simulink model "Simulation"  (R2022b)
settings: Solver=ode1  StartTime=0.0  StopTime=Tf  FixedStep=t_step  RelTol=1e-3
undefined symbols (not defined in the file or in its folder): F, Im, Kd, Kp, kr, lx, ly, lz, mm, qt, rho, t_step
libraries: slpidlib x1
settings Model: Creator=vincenzo  LastModifiedBy=vincenzo

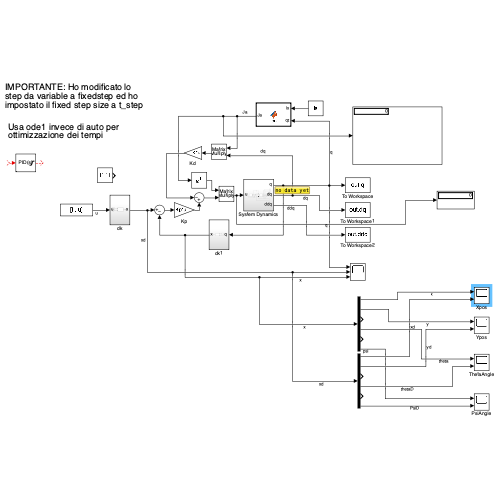
[thumbnail: Simulink's stored preview of the top-level diagram]
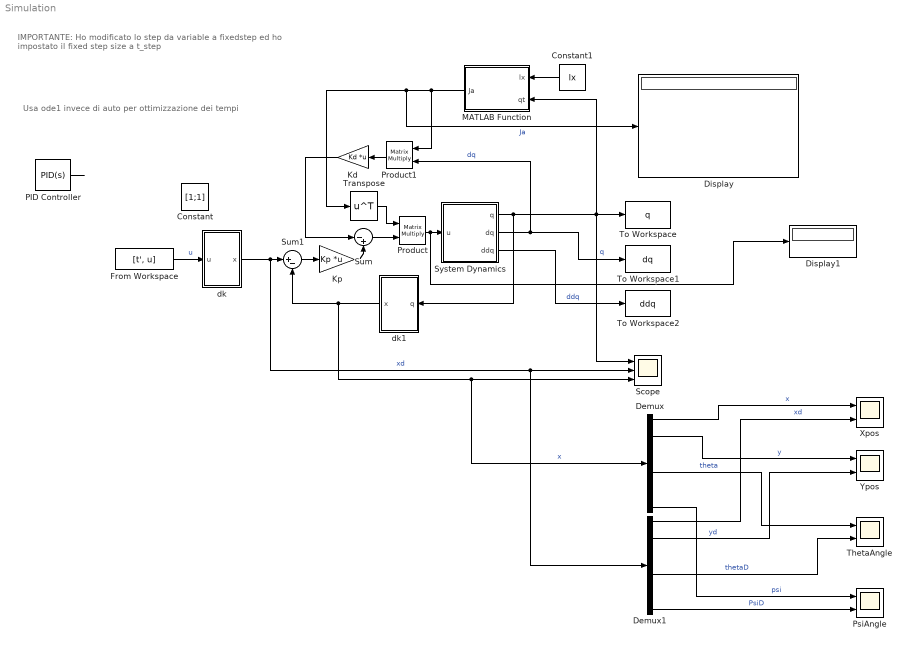
== system Simulation ==
  note: Usa ode1 invece di auto per ottimizzazione dei tempi
  note: IMPORTANTE: Ho modificato lo step da variable a fixedstep ed ho impostato il fixed step size a t_step
  Constant : Constant  Value=[1;1]
  Constant1 : Constant  Value=lx
  Demux : Demux  Outputs=6
  Demux1 : Demux  Outputs=6
  Display : Display
  Display1 : Display
  From Workspace : FromWorkspace  VariableName=[t', u]  OutDataTypeStr=double  SampleTime=t_step
  Kd : Gain  Gain=Kd  Multiplication=Matrix(K*u)
  Kp : Gain  Gain=Kp  Multiplication=Matrix(K*u)
  MATLAB Function : MATLAB Function  TreatAsAtomicUnit=on
  PID Controller : slpidlib/PID Controller  Controller=PID  Form=Parallel  TimeDomain=Continuous-time  UseExternalTs=off  SampleTime=-1  IntegratorMethod=Forward Euler  FilterMethod=Forward Euler  ControllerParametersSource=internal  P=1/100  I=0  UseKiTs=off  D=0  N=100  UseFilter=on  TunerSelectOption=Transfer Function Based (PID Tuner App)  InitialConditionSource=internal  InitialConditionForIntegrator=0  InitialConditionForFilter=0  DifferentiatorICPrevScaledInput=0  ExternalReset=none  TrackingMode=off  Kt=1  LimitOutput=on  SatLimitsSource=internal  UpperSaturationLimit=4.5  LowerSaturationLimit=-4.5  LinearizeAsGain=on  AntiWindupMode=clamping  Kb=1  LimitIntegrator=off  UpperIntegratorSaturationLimit=inf  LowerIntegratorSaturationLimit=-inf  POutMin=[]  POutMax=[]  IOutMin=[]  IOutMax=[]  DOutMin=[]  DOutMax=[]  NOutMin=[]  NOutMax=[]  SumOutMin=[]  SumOutMax=[]  SaturationOutMin=[]  SaturationOutMax=[]  PParamMin=[]  PParamMax=[]  IParamMin=[]  IParamMax=[]  DParamMin=[]  DParamMax=[]  NParamMin=[]  NParamMax=[]  KbParamMin=[]  KbParamMax=[]  KtParamMin=[]  KtParamMax=[]  KbOutMin=[]  KbOutMax=[]  KtOutMin=[]  KtOutMax=[]  IntegratorOutMin=[]  IntegratorOutMax=[]  FilterOutMin=[]  FilterOutMax=[]  SumI1OutMin=[]  SumI1OutMax=[]  SumI2OutMin=[]  SumI2OutMax=[]  SumI3OutMin=[]  SumI3OutMax=[]  SumI4OutMin=[]  SumI4OutMax=[]  SumDOutMin=[]  SumDOutMax=[]  DifferentiatorOutMin=[]  DifferentiatorOutMax=[]  FilterDiffOutCoefMin=[]  FilterDiffOutCoefMax=[]  ReciprocalOutMin=[]  ReciprocalOutMax=[]  SumDenOutMin=[]  SumDenOutMax=[]  SumNumOutMin=[]  SumNumOutMax=[]  DivideOutMin=[]  DivideOutMax=[]  UdiffTsProdOutMin=[]  UdiffTsProdOutMax=[]  NTsProdOutMin=[]  NTsProdOutMax=[]  UintegralTsProdOutMin=[]  UintegralTsProdOutMax=[]  UngainTsProdOutMin=[]  UngainTsProdOutMax=[]  ClampingZeroOutDataTypeStr=Inherit: Inherit via back propagation  ClampingZeroOutMin=[]  ClampingZeroOutMax=[]  FilterDenConstantOutDataTypeStr=Inherit: Inherit via back propagation  FilterDenConstantOutMin=[]  FilterDenConstantOutMax=[]  PCopyOutDataTypeStr=Inherit: Inherit via back propagation  PCopyOutMin=[]  PCopyOutMax=[]  NCopyOutDataTypeStr=Inherit: Inherit via back propagation  NCopyOutMin=[]  NCopyOutMax=[]  IntegratorContinuousStateAttributes=''  IntegratorStateMustResolveToSignalObject=off  IntegratorRTWStateStorageClass=Auto  FilterContinuousStateAttributes=''  FilterStateMustResolveToSignalObject=off  FilterRTWStateStorageClass=Auto  ParallelPVariant=InternalParameters  IdealPVariant=Disabled  IVariant=InternalParameters  DVariant=InternalParameters  IntegratorVariant=Continuous  SatVariant=Enabled  AWVariant=ContClampingParallel  PCopyVariant=Disabled  TRVariant=Disabled  FdbkBlocksVariant=Forward  IdealPFdbkVariant=Disabled  SatFdbkVariant=Disabled  DerivativeFilterVariant=ContFilter  NVariant=InternalParameters  NCopyVariant=Disabled  FilterICVariant=InternalICsFilter  IntegratorICVariant=InternalICs  ExternalResetVariant=Disabled  TRSumVariant=Passthrough  SumFdbkVariant=Disabled  SumVariant=Sum_PID  TsampFilterVariant=InternalTs  TsampNgainVariant=Passthrough  TsampIntegralVariant=Passthrough  ExternalSaturationOutDataTypeStr=Inherit: Same as second input
  Product : Product  Multiplication=Matrix(*)
  Product1 : Product  Multiplication=Matrix(*)
  PsiAngle : Scope  NumInputPorts=2
  Scope : Scope  NumInputPorts=3
  Sum : Sum  Inputs=|-+
  Sum1 : Sum  Inputs=|+-
  System Dynamics : Subsystem
  ThetaAngle : Scope  NumInputPorts=2
  To Workspace : ToWorkspace  VariableName=q  SampleTime=-1
      settings: Save2DSignal=2-D array (concatenate along first dimension)
  To Workspace1 : ToWorkspace  VariableName=dq  SampleTime=-1
      settings: Save2DSignal=2-D array (concatenate along first dimension)
  To Workspace2 : ToWorkspace  VariableName=ddq  SampleTime=-1
      settings: Save2DSignal=2-D array (concatenate along first dimension)
  Transpose : Math  Operator=transpose
  Xpos : Scope  NumInputPorts=2
  Ypos : Scope  NumInputPorts=2
  dk : Subsystem
  dk1 : Subsystem
  wires:
  ? -> PID Controller/1
  System Dynamics/1(q) -> dk1/1(q), Scope/1, To Workspace/1, MATLAB Function/2(qt)  "q"
  PID Controller/1 -> ?
  System Dynamics/2(dq) -> Product1/2, To Workspace1/1  "dq"
  System Dynamics/3(ddq) -> To Workspace2/1  "ddq"
  Sum1/1 -> Kp/1
  Kp/1 -> Sum/2
  Sum/1 -> Product/2
  Kd/1 -> Sum/1
  Product/1 -> Display1/1, System Dynamics/1(u)
  MATLAB Function/1(Ja) -> Product1/1, Display/1, Transpose/1  "Ja"
  Transpose/1 -> Product/1
  Constant1/1 -> MATLAB Function/1(lx)
  Product1/1 -> Kd/1
  dk/1(x) -> Demux1/1, Scope/2, Sum1/1  "xd"
  From Workspace/1 -> dk/1(u)  "u"
  dk1/1(x) -> Demux/1, Scope/3, Sum1/2  "x"
  Demux/1 -> Xpos/1  "x"
  Demux1/1 -> Xpos/2  "xd"
  Demux/2 -> Ypos/1  "y"
  Demux1/2 -> Ypos/2  "yd"
  Demux/4 -> ThetaAngle/1  "theta"
  Demux1/4 -> ThetaAngle/2  "thetaD"
  Demux1/6 -> PsiAngle/2  "PsiD"
  Demux/6 -> PsiAngle/1  "psi"

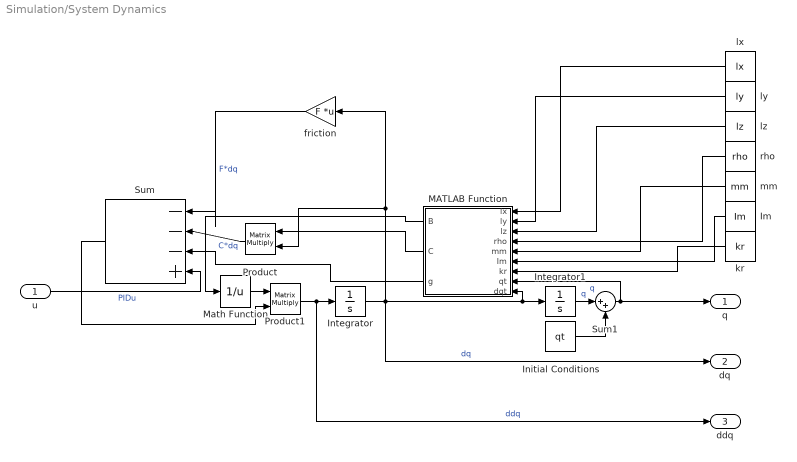
== system Simulation/System Dynamics ==
  u : Inport
  Im : Constant  Value=Im
  Initial Conditions : Constant  Value=qt
  Integrator : Integrator  InitialCondition=[0; 0]
  Integrator1 : Integrator  InitialCondition=[0;0]
  MATLAB Function : MATLAB Function  TreatAsAtomicUnit=on
  Math Function : Math  Operator=reciprocal
  Product : Product  Multiplication=Matrix(*)
  Product1 : Product  Multiplication=Matrix(*)
  Sum : Sum  Inputs=|---+
  Sum1 : Sum  Inputs=|++
  friction : Gain  Gain=F  Multiplication=Matrix(K*u)
  kr : Constant  Value=kr
  lx : Constant  Value=lx
  ly : Constant  Value=ly
  lz : Constant  Value=lz
  mm : Constant  Value=mm
  rho : Constant  Value=rho
  q : Outport
  dq : Outport  Port=2
  ddq : Outport  Port=3
  wires:
  Sum/1 -> Product1/2
  friction/1 -> Sum/1  "F*dq"
  MATLAB Function/1(B) -> Math Function/1
  Sum1/1 -> MATLAB Function/8(qt), q/1  "q"
  lx/1 -> MATLAB Function/1(lx)
  MATLAB Function/2(C) -> Product/1
  Product/1 -> Sum/2  "C*dq"
  Math Function/1 -> Product1/1
  ly/1 -> MATLAB Function/2(ly)
  Integrator/1 -> dq/1, Integrator1/1, MATLAB Function/9(dqt), Product/2, friction/1  "dq"
  Product1/1 -> ddq/1, Integrator/1  "ddq"
  MATLAB Function/3(g) -> Sum/3
  lz/1 -> MATLAB Function/3(lz)
  mm/1 -> MATLAB Function/5(mm)
  kr/1 -> MATLAB Function/7(kr)
  rho/1 -> MATLAB Function/4(rho)
  Im/1 -> MATLAB Function/6(Im)
  u/1 -> Sum/4  "PIDu"
  Integrator1/1 -> Sum1/1  "q"
  Initial Conditions/1 -> Sum1/2

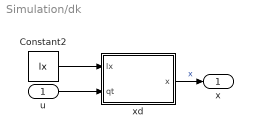
== system Simulation/dk ==
  u : Inport
  Constant2 : Constant  Value=lx
  xd : MATLAB Function  TreatAsAtomicUnit=on
  x : Outport
  wires:
  Constant2/1 -> xd/1(lx)
  u/1 -> xd/2(qt)
  xd/1(x) -> x/1  "x"

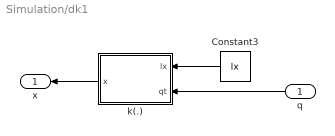
== system Simulation/dk1 ==
  q : Inport
  Constant3 : Constant  Value=lx
  k(.) : MATLAB Function  TreatAsAtomicUnit=on
  x : Outport
  wires:
  Constant3/1 -> k(.)/1(lx)
  q/1 -> k(.)/2(qt)
  k(.)/1(x) -> x/1

== matlab function Simulation/MATLAB Function ==
  data: lx input; Ja output; qt input
function Ja = fcn(lx, qt)
coder.extrinsic("jacobianFnc");
Ja = zeros(6,2);
Ja = jacobianFnc(lx, qt);

== matlab function Simulation/System Dynamics/MATLAB Function ==
  data: lx input; ly input; lz input; rho input; mm input; Im input; kr input; qt input; B output; dqt input; C output; g output
function [B, C, g] = fcn(lx, ly, lz, rho, mm, Im, kr, qt, dqt)
coder.extrinsic('generateBCg');
B = zeros(2);
C = zeros(2);
g = zeros(2,1);
[B, C, g] = generateBCg(lx, ly, lz, rho, mm, Im, kr, qt, dqt);

== matlab function Simulation/dk1/k(.) ==
  data: lx input; qt input; x output
function x = fcn(lx, qt)
coder.extrinsic("directkinematics")
x = zeros(6,1);
x = directkinematics(lx, qt);

== matlab function Simulation/dk/xd ==
  data: lx input; qt input; x output
function x = fcn(lx, qt)
coder.extrinsic("directkinematics")
x = zeros(6,1);
x = directkinematics(lx, qt);
